simulink model "robot_2015"  (R2015b)
(part 17 of 148)

  Cylindrical9/LConn1 -- hex_bolt_gradeb_iso_243_RIGID/RConn1
  Cylindrical9/RConn1 -- hex_nut_style_1_gradeab_iso_156_RIGID/LConn2
  Cylindrical10/LConn1 -- hex_bolt_gradeb_iso_247_RIGID/RConn1
  Cylindrical10/RConn1 -- hex_nut_style_1_gradeab_iso_158_RIGID/LConn2
  Cylindrical11/LConn1 -- hex_bolt_gradeb_iso_209_RIGID/RConn1
  Planar3/LConn1 -- hip_joint_casin_2_RIGID/RConn5
  Cylindrical11/RConn1 -- hex_nut_style_1_gradeab_iso_161_RIGID/LConn2
  Cylindrical12/LConn1 -- hex_bolt_gradeb_iso_211_RIGID/RConn1
  Cylindrical12/RConn1 -- hex_nut_style_1_gradeab_iso_162_RIGID/LConn1
  Cylindrical13/LConn1 -- hex_bolt_gradeb_iso_208_RIGID/RConn1
  Cylindrical13/RConn1 -- hex_nut_style_1_gradeab_iso_163_RIGID/LConn2
  Cylindrical14/LConn1 -- hex_bolt_gradeb_iso_249_RIGID/RConn1
  Cylindrical14/RConn1 -- hex_nut_style_1_gradeab_iso_164_RIGID/LConn2
  Cylindrical15/LConn1 -- hex_bolt_gradeb_iso_254_RIGID/RConn1
  Cylindrical15/RConn1 -- hex_nut_style_1_gradeab_iso_165_RIGID/LConn2
  Cylindrical16/LConn1 -- hex_bolt_gradeb_iso_253_RIGID/RConn1
  Planar3/RConn1 -- hex_nut_style_1_gradeab_iso_258_RIGID/LConn2
  Cylindrical16/RConn1 -- hex_nut_style_1_gradeab_iso_166_RIGID/LConn1
  Cylindrical17/LConn1 -- hex_bolt_gradeb_iso_210_RIGID/RConn1
  Cylindrical17/RConn1 -- hex_nut_style_1_gradeab_iso_167_RIGID/LConn2
  Cylindrical18/LConn1 -- hex_bolt_gradeb_iso_252_RIGID/RConn1
  Cylindrical18/RConn1 -- hex_nut_style_1_gradeab_iso_168_RIGID/LConn1
  Cylindrical19/LConn1 -- hex_bolt_gradeb_iso_251_RIGID/RConn1
  Cylindrical19/RConn1 -- hex_nut_style_1_gradeab_iso_169_RIGID/LConn2
  Cylindrical20/LConn1 -- hex_bolt_gradeb_iso_250_RIGID/RConn1
  Cylindrical20/RConn1 -- hex_nut_style_1_gradeab_iso_170_RIGID/LConn2
  Cylindrical21/LConn1 -- hex_bolt_gradeb_iso_206_RIGID/RConn1
  Planar4/LConn1 -- hip_joint_casin_2_RIGID/RConn3
  Cylindrical21/RConn1 -- hex_nut_style_1_gradeab_iso_171_RIGID/LConn1
  Cylindrical22/LConn1 -- hex_bolt_gradeb_iso_207_RIGID/RConn1
  Cylindrical22/RConn1 -- hex_nut_style_1_gradeab_iso_172_RIGID/LConn1
  Cylindrical23/LConn1 -- hex_bolt_gradeb_iso_220_RIGID/RConn1
  Cylindrical23/RConn1 -- hex_nut_style_1_gradeab_iso_185_RIGID/LConn1
  Cylindrical24/LConn1 -- hex_bolt_gradeb_iso_221_RIGID/RConn1
  Cylindrical24/RConn1 -- hex_nut_style_1_gradeab_iso_186_RIGID/LConn2
  Cylindrical25/LConn1 -- hex_bolt_gradeb_iso_222_RIGID/RConn1
  Cylindrical25/RConn1 -- hex_nut_style_1_gradeab_iso_187_RIGID/LConn2
  Cylindrical26/LConn1 -- hex_bolt_gradeb_iso_223_RIGID/RConn1
  Planar4/RConn1 -- hex_nut_style_1_gradeab_iso_259_RIGID/LConn2
  Cylindrical26/RConn1 -- hex_nut_style_1_gradeab_iso_188_RIGID/LConn2
  Cylindrical27/LConn1 -- hex_bolt_gradeb_iso_218_RIGID/RConn1
  Cylindrical27/RConn1 -- hex_nut_style_1_gradeab_iso_189_RIGID/LConn1
  Cylindrical28/LConn1 -- hex_bolt_gradeb_iso_219_RIGID/RConn1
  Cylindrical28/RConn1 -- hex_nut_style_1_gradeab_iso_190_RIGID/LConn1
  Cylindrical29/LConn1 -- hex_bolt_gradeb_iso_257_RIGID/RConn1
  Cylindrical29/RConn1 -- hex_nut_style_1_gradeab_iso_191_RIGID/LConn2
  Cylindrical30/LConn1 -- hex_bolt_gradeb_iso_258_RIGID/RConn1
  Cylindrical30/RConn1 -- hex_nut_style_1_gradeab_iso_192_RIGID/LConn2
  Cylindrical31/LConn1 -- hex_bolt_gradeb_iso_259_RIGID/RConn1
  Revolute1/RConn1 -- hex_nut_style_1_gradeab_iso_249_RIGID/LConn1
  Planar5/LConn1 -- hip_joint_casin_2_RIGID/RConn6
  Cylindrical31/RConn1 -- hex_nut_style_1_gradeab_iso_193_RIGID/LConn2
  Cylindrical32/LConn1 -- hex_bolt_gradeb_iso_260_RIGID/RConn1
  Cylindrical32/RConn1 -- hex_nut_style_1_gradeab_iso_194_RIGID/LConn2
  Cylindrical33/LConn1 -- hex_bolt_gradeb_iso_255_RIGID/RConn1
  Cylindrical33/RConn1 -- hex_nut_style_1_gradeab_iso_195_RIGID/LConn1
  Cylindrical34/LConn1 -- hex_bolt_gradeb_iso_256_RIGID/RConn1
  Cylindrical34/RConn1 -- hex_nut_style_1_gradeab_iso_196_RIGID/LConn1
  Cylindrical35/LConn1 -- hex_bolt_gradeb_iso_235_RIGID/RConn1
  Cylindrical35/RConn1 -- hex_nut_style_1_gradeab_iso_197_RIGID/LConn1
  Cylindrical36/LConn1 -- hex_bolt_gradeb_iso_230_RIGID/RConn1
  Planar5/RConn1 -- hex_nut_style_1_gradeab_iso_260_RIGID/LConn1
  Cylindrical36/RConn1 -- hex_nut_style_1_gradeab_iso_199_RIGID/LConn2
  Cylindrical37/LConn1 -- hex_bolt_gradeb_iso_234_RIGID/RConn1
  Cylindrical37/RConn1 -- hex_nut_style_1_gradeab_iso_201_RIGID/LConn1
  Cylindrical38/LConn1 -- hex_bolt_gradeb_iso_233_RIGID/RConn1
  Cylindrical38/RConn1 -- hex_nut_style_1_gradeab_iso_204_RIGID/LConn2
  Cylindrical39/LConn1 -- hex_bolt_gradeb_iso_232_RIGID/RConn1
  Cylindrical39/RConn1 -- hex_nut_style_1_gradeab_iso_205_RIGID/LConn1
  Cylindrical40/LConn1 -- hex_bolt_gradeb_iso_231_RIGID/RConn1
  Cylindrical40/RConn1 -- hex_nut_style_1_gradeab_iso_206_RIGID/LConn1
  Cylindrical41/LConn1 -- hex_bolt_gradeb_iso_268_RIGID/RConn1
  Revolute14/LConn1 -- hip_joint_casin_2_RIGID/RConn2
  Cylindrical41/RConn1 -- hex_nut_style_1_gradeab_iso_215_RIGID/LConn2
  Cylindrical42/LConn1 -- hex_bolt_gradeb_iso_267_RIGID/RConn1
  Cylindrical42/RConn1 -- hex_nut_style_1_gradeab_iso_216_RIGID/LConn1
  Cylindrical43/LConn1 -- hex_bolt_gradeb_iso_271_RIGID/RConn1
  Cylindrical43/RConn1 -- hex_nut_style_1_gradeab_iso_217_RIGID/LConn2
  Cylindrical44/LConn1 -- hex_bolt_gradeb_iso_272_RIGID/RConn1
  Cylindrical44/RConn1 -- hex_nut_style_1_gradeab_iso_218_RIGID/LConn1
  Cylindrical45/LConn1 -- hex_bolt_gradeb_iso_270_RIGID/RConn1
  Cylindrical45/RConn1 -- hex_nut_style_1_gradeab_iso_219_RIGID/LConn1
  Cylindrical46/LConn1 -- hex_bolt_gradeb_iso_269_RIGID/RConn1
  Revolute14/RConn1 -- hex_bolt_gradeb_iso_206_RIGID/LConn1
  Cylindrical46/RConn1 -- hex_nut_style_1_gradeab_iso_220_RIGID/LConn2
  Cylindrical47/LConn1 -- hex_bolt_gradeb_iso_160_RIGID/RConn1
  Cylindrical47/RConn1 -- hex_nut_style_1_gradeab_iso_222_RIGID/LConn1
  Cylindrical48/LConn1 -- hex_bolt_gradeb_iso_161_RIGID/RConn1
  Cylindrical48/RConn1 -- hex_nut_style_1_gradeab_iso_223_RIGID/LConn1
  Cylindrical49/LConn1 -- hex_bolt_gradeb_iso_162_RIGID/RConn1
  Cylindrical49/RConn1 -- hex_nut_style_1_gradeab_iso_224_RIGID/LConn1
  Cylindrical50/LConn1 -- hex_bolt_gradeb_iso_157_RIGID/RConn1
  Cylindrical50/RConn1 -- hex_nut_style_1_gradeab_iso_225_RIGID/LConn1
  Cylindrical51/LConn1 -- hex_bolt_gradeb_iso_158_RIGID/RConn1
  Revolute15/LConn1 -- hip_joint_casin_2_RIGID/RConn1
  Cylindrical51/RConn1 -- hex_nut_style_1_gradeab_iso_226_RIGID/LConn1
  Cylindrical52/LConn1 -- hex_bolt_gradeb_iso_159_RIGID/RConn1
  Cylindrical52/RConn1 -- hex_nut_style_1_gradeab_iso_227_RIGID/LConn1
  Cylindrical53/LConn1 -- hex_bolt_gradeb_iso_171_RIGID/RConn1
  Cylindrical53/RConn1 -- hex_nut_style_1_gradeab_iso_240_RIGID/LConn2
  Cylindrical54/LConn1 -- hex_bolt_gradeb_iso_170_RIGID/RConn1
  Cylindrical54/RConn1 -- hex_nut_style_1_gradeab_iso_241_RIGID/LConn2
  Cylindrical55/LConn1 -- hex_bolt_gradeb_iso_174_RIGID/RConn1
  Cylindrical55/RConn1 -- hex_nut_style_1_gradeab_iso_242_RIGID/LConn1
  Cylindrical56/LConn1 -- hex_bolt_gradeb_iso_173_RIGID/RConn1
  Revolute15/RConn1 -- hex_bolt_gradeb_iso_207_RIGID/LConn1
  Cylindrical56/RConn1 -- hex_nut_style_1_gradeab_iso_243_RIGID/LConn2
  Cylindrical57/LConn1 -- hex_bolt_gradeb_iso_172_RIGID/RConn1
  Cylindrical57/RConn1 -- hex_nut_style_1_gradeab_iso_244_RIGID/LConn1
  Cylindrical58/LConn1 -- hex_bolt_gradeb_iso_169_RIGID/RConn1
  Cylindrical58/RConn1 -- hex_nut_style_1_gradeab_iso_248_RIGID/LConn2
  Cylindrical59/LConn1 -- hex_bolt_gradeb_iso_147_RIGID/RConn1
  Cylindrical59/RConn1 -- hex_nut_style_1_gradeab_iso_255_RIGID/LConn1
  Cylindrical60/LConn1 -- hex_bolt_gradeb_iso_148_RIGID/RConn1
  Cylindrical60/RConn1 -- hex_nut_style_1_gradeab_iso_256_RIGID/LConn2
  Cylindrical61/LConn1 -- hex_bolt_gradeb_iso_146_RIGID/RConn1
  Revolute16/LConn1 -- hip_joint_casin_2_RIGID/RConn12
  Cylindrical61/RConn1 -- hex_nut_style_1_gradeab_iso_257_RIGID/LConn2
  Cylindrical62/LConn1 -- hex_bolt_gradeb_iso_150_RIGID/RConn1
  Cylindrical62/RConn1 -- hex_nut_style_1_gradeab_iso_258_RIGID/LConn1
  Cylindrical63/LConn1 -- hex_bolt_gradeb_iso_149_RIGID/RConn1
  Cylindrical63/RConn1 -- hex_nut_style_1_gradeab_iso_259_RIGID/LConn1
  Cylindrical64/LConn1 -- hex_bolt_gradeb_iso_145_RIGID/RConn1
  Cylindrical64/RConn1 -- hex_nut_style_1_gradeab_iso_260_RIGID/LConn2
  Cylindrical65/LConn1 -- hex_bolt_gradeb_iso_181_RIGID/RConn1
  Cylindrical65/RConn1 -- hex_nut_style_1_gradeab_iso_267_RIGID/LConn2
  Cylindrical66/LConn1 -- hex_bolt_gradeb_iso_184_RIGID/RConn1
  Revolute16/RConn1 -- hex_bolt_gradeb_iso_208_RIGID/LConn1
  Cylindrical66/RConn1 -- hex_nut_style_1_gradeab_iso_268_RIGID/LConn1
  Cylindrical67/LConn1 -- hex_bolt_gradeb_iso_185_RIGID/RConn1
  Cylindrical67/RConn1 -- hex_nut_style_1_gradeab_iso_269_RIGID/LConn1
  Cylindrical68/LConn1 -- hex_bolt_gradeb_iso_186_RIGID/RConn1
  Cylindrical68/RConn1 -- hex_nut_style_1_gradeab_iso_270_RIGID/LConn1
  Cylindrical69/LConn1 -- hex_bolt_gradeb_iso_182_RIGID/RConn1
  Cylindrical69/RConn1 -- hex_nut_style_1_gradeab_iso_271_RIGID/LConn1
  Cylindrical70/LConn1 -- hex_bolt_gradeb_iso_183_RIGID/RConn1
  Cylindrical70/RConn1 -- hex_nut_style_1_gradeab_iso_272_RIGID/LConn1
  Cylindrical71/LConn1 -- hex_bolt_gradeb_iso_195_RIGID/RConn1
  Revolute17/LConn1 -- hip_joint_casin_2_RIGID/RConn11
  Cylindrical71/RConn1 -- hex_nut_style_1_gradeab_iso_279_RIGID/LConn1
  Cylindrical72/LConn1 -- hex_bolt_gradeb_iso_194_RIGID/RConn1
  Cylindrical72/RConn1 -- hex_nut_style_1_gradeab_iso_280_RIGID/LConn2
  Cylindrical73/LConn1 -- hex_bolt_gradeb_iso_193_RIGID/RConn1
  Cylindrical73/RConn1 -- hex_nut_style_1_gradeab_iso_281_RIGID/LConn2
  Cylindrical74/LConn1 -- hex_bolt_gradeb_iso_198_RIGID/RConn1
  Cylindrical74/RConn1 -- hex_nut_style_1_gradeab_iso_282_RIGID/LConn1
  Cylindrical75/LConn1 -- hex_bolt_gradeb_iso_197_RIGID/RConn1
  Cylindrical75/RConn1 -- hex_nut_style_1_gradeab_iso_283_RIGID/LConn1
  Cylindrical76/LConn1 -- hex_bolt_gradeb_iso_196_RIGID/RConn1
  Revolute17/RConn1 -- hex_bolt_gradeb_iso_209_RIGID/LConn1
  Cylindrical76/RConn1 -- hex_nut_style_1_gradeab_iso_284_RIGID/LConn1
  Rectangular1/LConn1 -- SEA_system_1_RIGID/RConn1
  Rectangular1/RConn1 -- lower_leg_main_1_RIGID/LConn2
  Revolute111/LConn1 -- lower_leg_main_1_RIGID/RConn12
  Revolute111/RConn1 -- hex_bolt_gradeb_iso_193_RIGID/LConn1
  Revolute112/LConn1 -- lower_leg_main_1_RIGID/RConn10
  Revolute112/RConn1 -- hex_bolt_gradeb_iso_194_RIGID/LConn1
  Revolute113/LConn1 -- lower_leg_main_1_RIGID/RConn7
  Revolute113/RConn1 -- hex_bolt_gradeb_iso_195_RIGID/LConn1
  Revolute114/LConn1 -- lower_leg_main_1_RIGID/RConn6
  Revolute2/LConn1 -- hip_joint_casin_1_RIGID/RConn7
  Revolute18/LConn1 -- hip_joint_casin_2_RIGID/RConn10
  Revolute114/RConn1 -- hex_bolt_gradeb_iso_196_RIGID/LConn1
  Revolute115/LConn1 -- lower_leg_main_1_RIGID/RConn5
  Revolute115/RConn1 -- hex_bolt_gradeb_iso_197_RIGID/LConn1
  Revolute116/LConn1 -- lower_leg_main_1_RIGID/RConn4
  Revolute116/RConn1 -- hex_bolt_gradeb_iso_198_RIGID/LConn1
  Revolute117/LConn1 -- lower_leg_main_1_RIGID/RConn3
  Revolute117/RConn1 -- hex_bolt_gradeb_iso_199_RIGID/LConn1
  Revolute118/LConn1 -- lower_leg_main_1_RIGID/RConn2
  Revolute118/RConn1 -- hex_bolt_gradeb_iso_200_RIGID/LConn1
  Revolute119/LConn1 -- lower_leg_main_1_RIGID/RConn1
  Revolute18/RConn1 -- hex_bolt_gradeb_iso_210_RIGID/LConn1
  Revolute119/RConn1 -- hex_bolt_gradeb_iso_201_RIGID/LConn1
  Revolute120/LConn1 -- lower_leg_main_1_RIGID/RConn11
  Revolute120/RConn1 -- hex_bolt_gradeb_iso_202_RIGID/LConn1
  Revolute121/LConn1 -- lower_leg_main_1_RIGID/RConn9
  Revolute121/RConn1 -- hex_bolt_gradeb_iso_203_RIGID/LConn1
  Revolute122/LConn1 -- lower_leg_main_1_RIGID/RConn8
  Revolute122/RConn1 -- hex_bolt_gradeb_iso_204_RIGID/LConn1
  Cylindrical77/LConn1 -- motor_axle_1_RIGID/RConn2
  Cylindrical77/RConn1 -- upper_leg_casin_2_RIGID/LConn2
  Revolute123/LConn1 -- motor_body_1_RIGID/RConn1
  Revolute19/LConn1 -- hip_joint_casin_2_RIGID/RConn8
  Revolute123/RConn1 -- upper_leg_casin_2_RIGID/LConn3
  Revolute124/LConn1 -- upper_leg_casin_2_RIGID/RConn7
  Revolute124/RConn1 -- hex_bolt_gradeb_iso_243_RIGID/LConn1
  Revolute125/LConn1 -- upper_leg_casin_2_RIGID/RConn6
  Revolute125/RConn1 -- hex_bolt_gradeb_iso_244_RIGID/LConn1
  Revolute126/LConn1 -- upper_leg_casin_2_RIGID/RConn5
  Revolute126/RConn1 -- hex_bolt_gradeb_iso_245_RIGID/LConn1
  Revolute127/LConn1 -- upper_leg_casin_2_RIGID/RConn4
  Revolute127/RConn1 -- hex_bolt_gradeb_iso_246_RIGID/LConn1
  Revolute128/LConn1 -- upper_leg_casin_2_RIGID/RConn3
  Revolute19/RConn1 -- hex_bolt_gradeb_iso_211_RIGID/LConn1
  Revolute128/RConn1 -- hex_bolt_gradeb_iso_247_RIGID/LConn1
  Revolute129/LConn1 -- upper_leg_casin_2_RIGID/RConn2
  Revolute129/RConn1 -- hex_bolt_gradeb_iso_248_RIGID/LConn1
  Prismatic4/LConn1 -- upper_leg_casin_2_RIGID/RConn1
  Prismatic4/RConn1 -- upper_leg_cap_7_RIGID/LConn2
  motor_body_2_RIGID/LConn1 -- upper_leg_casin_3_RIGID/LConn4
  Planar44/LConn1 -- upper_leg_casin_3_RIGID/RConn8
  Planar44/RConn1 -- hex_nut_style_1_gradeab_iso_222_RIGID/LConn2
  Planar45/LConn1 -- upper_leg_casin_3_RIGID/RConn7
  Planar45/RConn1 -- hex_nut_style_1_gradeab_iso_223_RIGID/LConn2
  Lower_joint_cap_1_RIGID/RConn6 -- Revolute20/LConn1
  Planar46/LConn1 -- upper_leg_casin_3_RIGID/RConn6
  Planar46/RConn1 -- hex_nut_style_1_gradeab_iso_224_RIGID/LConn2
  Planar47/LConn1 -- upper_leg_casin_3_RIGID/RConn5
  Planar47/RConn1 -- hex_nut_style_1_gradeab_iso_225_RIGID/LConn2
  Planar48/LConn1 -- upper_leg_casin_3_RIGID/RConn4
  Planar48/RConn1 -- hex_nut_style_1_gradeab_iso_226_RIGID/LConn2
  Planar49/LConn1 -- upper_leg_casin_3_RIGID/RConn3
  Planar49/RConn1 -- hex_nut_style_1_gradeab_iso_227_RIGID/LConn2
  Revolute130/LConn1 -- upper_leg_casin_3_RIGID/RConn2
  Revolute130/RConn1 -- hex_bolt_gradeb_iso_261_RIGID/LConn1
  Revolute20/RConn1 -- hex_nut_style_1_gradeab_iso_145_RIGID/LConn1
  Revolute131/LConn1 -- upper_leg_casin_3_RIGID/RConn1
  Revolute131/RConn1 -- hex_bolt_gradeb_iso_262_RIGID/LConn1
  Revolute132/LConn1 -- upper_leg_casin_3_RIGID/RConn12
  Revolute132/RConn1 -- hex_bolt_gradeb_iso_263_RIGID/LConn1
  Revolute133/LConn1 -- upper_leg_casin_3_RIGID/RConn11
  Revolute133/RConn1 -- hex_bolt_gradeb_iso_264_RIGID/LConn1
  Revolute134/LConn1 -- upper_leg_casin_3_RIGID/RConn10
  Revolute134/RConn1 -- hex_bolt_gradeb_iso_265_RIGID/LConn1
  Revolute135/LConn1 -- upper_leg_casin_3_RIGID/RConn9
  Revolute135/RConn1 -- hex_bolt_gradeb_iso_266_RIGID/LConn1
  Lower_joint_cap_1_RIGID/RConn5 -- Revolute21/LConn1
  Prismatic5/LConn1 -- upper_leg_cap_3_RIGID/RConn1
  Prismatic5/RConn1 -- upper_leg_casin_3_RIGID/LConn2
  Revolute136/LConn1 -- upper_leg_casin_4_RIGID/RConn11
  Revolute136/RConn1 -- hex_nut_style_1_gradeab_iso_228_RIGID/LConn1
  Revolute137/LConn1 -- upper_leg_casin_4_RIGID/RConn8
  Revolute137/RConn1 -- hex_nut_style_1_gradeab_iso_230_RIGID/LConn1
  Revolute138/LConn1 -- upper_leg_casin_4_RIGID/RConn7
  Revolute138/RConn1 -- hex_nut_style_1_gradeab_iso_231_RIGID/LConn1
  Revolute139/LConn1 -- upper_leg_casin_4_RIGID/RConn6
  Revolute139/RConn1 -- hex_nut_style_1_gradeab_iso_232_RIGID/LConn1
  Revolute21/RConn1 -- hex_nut_style_1_gradeab_iso_146_RIGID/LConn1
  Revolute140/LConn1 -- upper_leg_casin_4_RIGID/RConn5
  Revolute140/RConn1 -- hex_nut_style_1_gradeab_iso_233_RIGID/LConn1
  Revolute141/LConn1 -- upper_leg_casin_4_RIGID/RConn4
  Revolute141/RConn1 -- hex_bolt_gradeb_iso_255_RIGID/LConn1
  Revolute142/LConn1 -- upper_leg_casin_4_RIGID/RConn1
  Revolute142/RConn1 -- hex_bolt_gradeb_iso_256_RIGID/LConn1
  Revolute143/LConn1 -- upper_leg_casin_4_RIGID/RConn3
  Revolute143/RConn1 -- hex_bolt_gradeb_iso_257_RIGID/LConn1
  Revolute144/LConn1 -- upper_leg_casin_4_RIGID/RConn2
  Revolute144/RConn1 -- hex_bolt_gradeb_iso_258_RIGID/LConn1
  Lower_joint_cap_1_RIGID/RConn4 -- Revolute22/LConn1
  Revolute145/LConn1 -- upper_leg_casin_4_RIGID/RConn10
  Revolute145/RConn1 -- hex_bolt_gradeb_iso_259_RIGID/LConn1
  Revolute146/LConn1 -- upper_leg_casin_4_RIGID/RConn9
  Revolute146/RConn1 -- hex_bolt_gradeb_iso_260_RIGID/LConn1
  Prismatic6/LConn1 -- upper_leg_cap_4_RIGID/RConn1
  Prismatic6/RConn1 -- upper_leg_casin_4_RIGID/LConn2
  Cylindrical78/LConn1 -- motor_axle_3_RIGID/RConn2
  Cylindrical78/RConn1 -- upper_leg_casin_5_RIGID/LConn3
  Revolute147/LConn1 -- motor_body_3_RIGID/RConn1
  Revolute147/RConn1 -- upper_leg_casin_5_RIGID/LConn4
  Revolute22/RConn1 -- hex_nut_style_1_gradeab_iso_147_RIGID/LConn1
  upper_leg_casin_5_RIGID/LConn1 -- upperleg_1_RIGID/LConn5
  Planar50/LConn1 -- upper_leg_casin_5_RIGID/RConn5
  Planar50/RConn1 -- hex_nut_style_1_gradeab_iso_267_RIGID/LConn1
  Planar51/LConn1 -- upper_leg_casin_5_RIGID/RConn4
  Planar51/RConn1 -- hex_nut_style_1_gradeab_iso_268_RIGID/LConn2
  Planar52/LConn1 -- upper_leg_casin_5_RIGID/RConn3
  Planar52/RConn1 -- hex_nut_style_1_gradeab_iso_269_RIGID/LConn2
  Planar53/LConn1 -- upper_leg_casin_5_RIGID/RConn2
  Planar53/RConn1 -- hex_nut_style_1_gradeab_iso_270_RIGID/LConn2
  Planar54/LConn1 -- upper_leg_casin_5_RIGID/RConn1
  Revolute2/RConn1 -- hex_nut_style_1_gradeab_iso_250_RIGID/LConn1
  Lower_joint_cap_1_RIGID/RConn3 -- Revolute23/LConn1
  Planar54/RConn1 -- hex_nut_style_1_gradeab_iso_271_RIGID/LConn2
  Planar55/LConn1 -- upper_leg_casin_5_RIGID/RConn8
  Planar55/RConn1 -- hex_nut_style_1_gradeab_iso_272_RIGID/LConn2
  Revolute148/LConn1 -- upper_leg_casin_5_RIGID/RConn12
  Revolute148/RConn1 -- hex_bolt_gradeb_iso_273_RIGID/LConn1
  Revolute149/LConn1 -- upper_leg_casin_5_RIGID/RConn11
  Revolute149/RConn1 -- hex_bolt_gradeb_iso_274_RIGID/LConn1
  Revolute150/LConn1 -- upper_leg_casin_5_RIGID/RConn10
  Revolute150/RConn1 -- hex_bolt_gradeb_iso_275_RIGID/LConn1
  Revolute151/LConn1 -- upper_leg_casin_5_RIGID/RConn9
  Revolute23/RConn1 -- hex_nut_style_1_gradeab_iso_150_RIGID/LConn1
  Revolute151/RConn1 -- hex_bolt_gradeb_iso_276_RIGID/LConn1
  Revolute152/LConn1 -- upper_leg_casin_5_RIGID/RConn7
  Revolute152/RConn1 -- hex_bolt_gradeb_iso_277_RIGID/LConn1
  Revolute153/LConn1 -- upper_leg_casin_5_RIGID/RConn6
  Revolute153/RConn1 -- hex_bolt_gradeb_iso_278_RIGID/LConn1
  upper_leg_casin_6_RIGID/LConn1 -- upperleg_1_RIGID/LConn4
  Revolute154/LConn1 -- upper_leg_casin_6_RIGID/RConn10
  Revolute154/RConn1 -- hex_nut_style_1_gradeab_iso_261_RIGID/LConn1
  Revolute155/LConn1 -- upper_leg_casin_6_RIGID/RConn9
  Revolute155/RConn1 -- hex_nut_style_1_gradeab_iso_262_RIGID/LConn1
  Lower_joint_cap_1_RIGID/RConn2 -- Revolute24/LConn1
  Revolute156/LConn1 -- upper_leg_casin_6_RIGID/RConn7
  Revolute156/RConn1 -- hex_nut_style_1_gradeab_iso_263_RIGID/LConn1
  Revolute157/LConn1 -- upper_leg_casin_6_RIGID/RConn6
  Revolute157/RConn1 -- hex_nut_style_1_gradeab_iso_264_RIGID/LConn1
  Revolute158/LConn1 -- upper_leg_casin_6_RIGID/RConn5
  Revolute158/RConn1 -- hex_nut_style_1_gradeab_iso_265_RIGID/LConn1
  Revolute159/LConn1 -- upper_leg_casin_6_RIGID/RConn4
  Revolute159/RConn1 -- hex_nut_style_1_gradeab_iso_266_RIGID/LConn1
  Revolute160/LConn1 -- upper_leg_casin_6_RIGID/RConn1
  Revolute160/RConn1 -- hex_bolt_gradeb_iso_267_RIGID/LConn1
  Revolute24/RConn1 -- hex_nut_style_1_gradeab_iso_159_RIGID/LConn1
  Revolute161/LConn1 -- upper_leg_casin_6_RIGID/RConn13
  Revolute161/RConn1 -- hex_bolt_gradeb_iso_268_RIGID/LConn1
  Revolute162/LConn1 -- upper_leg_casin_6_RIGID/RConn12
  Revolute162/RConn1 -- hex_bolt_gradeb_iso_269_RIGID/LConn1
  Revolute163/LConn1 -- upper_leg_casin_6_RIGID/RConn2
  Revolute163/RConn1 -- hex_bolt_gradeb_iso_270_RIGID/LConn1
  Revolute164/LConn1 -- upper_leg_casin_6_RIGID/RConn11
  Revolute164/RConn1 -- hex_bolt_gradeb_iso_271_RIGID/LConn1
  Revolute165/LConn1 -- upper_leg_casin_6_RIGID/RConn3
  Revolute165/RConn1 -- hex_bolt_gradeb_iso_272_RIGID/LConn1
  Lower_joint_cap_1_RIGID/RConn1 -- Revolute25/LConn1
  Revolute166/LConn1 -- upper_leg_casin_7_RIGID/RConn6
  Revolute166/RConn1 -- hex_bolt_gradeb_iso_249_RIGID/LConn1
  Revolute167/LConn1 -- upper_leg_casin_7_RIGID/RConn5
  Revolute167/RConn1 -- hex_bolt_gradeb_iso_250_RIGID/LConn1
  Revolute168/LConn1 -- upper_leg_casin_7_RIGID/RConn4
  Revolute168/RConn1 -- hex_bolt_gradeb_iso_251_RIGID/LConn1
  Revolute169/LConn1 -- upper_leg_casin_7_RIGID/RConn3
  Revolute169/RConn1 -- hex_bolt_gradeb_iso_252_RIGID/LConn1
  Revolute170/LConn1 -- upper_leg_casin_7_RIGID/RConn1
  Revolute170/RConn1 -- hex_bolt_gradeb_iso_253_RIGID/LConn1
  Revolute25/RConn1 -- hex_nut_style_1_gradeab_iso_160_RIGID/LConn1
  Revolute171/LConn1 -- upper_leg_casin_7_RIGID/RConn2
  Revolute171/RConn1 -- hex_bolt_gradeb_iso_254_RIGID/LConn1
  Prismatic7/LConn1 -- upper_leg_cap_1_RIGID/RConn2
  Prismatic7/RConn1 -- upper_leg_casin_7_RIGID/LConn2
  Prismatic8/LConn1 -- motor_axle_1_RIGID/RConn1
  Prismatic8/RConn1 -- SEA_system_hip_1_RIGID/LConn2
  Rectangular2/LConn1 -- hip_1_RIGID/RConn25
  Rectangular2/RConn1 -- SEA_system_hip_1_RIGID/LConn1
  Lower_joint_casin_1_RIGID/RConn12 -- Prismatic9/LConn1
  Prismatic9/RConn1 -- beam_filler_1_RIGID/LConn1
  Ball_bearing_filler_2_RIGID/LConn1 -- Lower_joint_cap_1_RIGID/LConn1
  beam_filler_1_RIGID/LConn2 -- upperleg_1_RIGID/LConn3
  Lower_joint_casin_2_RIGID/LConn2 -- beam_filler_2_RIGID/LConn1
  beam_filler_2_RIGID/LConn2 -- upperleg_1_RIGID/LConn1
  Lower_joint_casin_5_RIGID/LConn3 -- beam_filler_3_RIGID/LConn1
  beam_filler_3_RIGID/LConn2 -- lower_leg_main_1_RIGID/LConn1
  Revolute172/LConn1 -- beam_filler_4_RIGID/RConn2
  Lower_joint_casin_3_RIGID/LConn2 -- Revolute172/RConn1
  Prismatic10/LConn1 -- beam_filler_4_RIGID/RConn1
  Prismatic10/RConn1 -- lower_leg_main_1_RIGID/LConn3
  Planar56/LConn1 -- upper_leg_cap_1_RIGID/RConn1
  Lower_joint_cap_2_RIGID/RConn6 -- Planar6/LConn1
  Planar56/RConn1 -- bearing_1_RIGID/LConn1
  Ball_bearing_filler_small_1_RIGID/LConn2 -- upper_leg_cap_1_RIGID/LConn1
  Planar57/LConn1 -- upper_leg_cap_2_RIGID/RConn6
  Planar57/RConn1 -- hex_nut_style_1_gradeab_iso_164_RIGID/LConn1
  Planar58/LConn1 -- upper_leg_cap_2_RIGID/RConn5
  Planar58/RConn1 -- hex_nut_style_1_gradeab_iso_165_RIGID/LConn1
  Planar59/LConn1 -- upper_leg_cap_2_RIGID/RConn2
  Planar59/RConn1 -- hex_nut_style_1_gradeab_iso_166_RIGID/LConn2
  Planar60/LConn1 -- upper_leg_cap_2_RIGID/RConn1
  Planar60/RConn1 -- hex_nut_style_1_gradeab_iso_168_RIGID/LConn2
  Planar6/RConn1 -- hex_nut_style_1_gradeab_iso_161_RIGID/LConn1
  Planar61/LConn1 -- upper_leg_cap_2_RIGID/RConn4
  Planar61/RConn1 -- hex_nut_style_1_gradeab_iso_169_RIGID/LConn1
  Planar62/LConn1 -- upper_leg_cap_2_RIGID/RConn3
  Planar62/RConn1 -- hex_nut_style_1_gradeab_iso_170_RIGID/LConn1
  Ball_bearing_filler_small_1_RIGID/LConn1 -- upper_leg_cap_2_RIGID/LConn1
  Revolute173/LConn1 -- bearing_3_RIGID/RConn1
  Revolute173/RConn1 -- upper_leg_cap_3_RIGID/LConn2
  Ball_bearing_filler_small_4_RIGID/LConn2 -- upper_leg_cap_3_RIGID/LConn1
  Revolute174/LConn1 -- upper_leg_cap_4_RIGID/RConn2
  Revolute174/RConn1 -- bearing_4_RIGID/LConn1
  Lower_joint_cap_2_RIGID/RConn3 -- Planar7/LConn1
  Ball_bearing_filler_small_3_RIGID/LConn2 -- upper_leg_cap_4_RIGID/LConn1
  Revolute175/LConn1 -- upper_leg_cap_5_RIGID/RConn6
  Revolute175/RConn1 -- hex_nut_style_1_gradeab_iso_198_RIGID/LConn1
  Revolute176/LConn1 -- upper_leg_cap_5_RIGID/RConn5
  Revolute176/RConn1 -- hex_nut_style_1_gradeab_iso_200_RIGID/LConn1
  Revolute177/LConn1 -- upper_leg_cap_5_RIGID/RConn4
  Revolute177/RConn1 -- hex_nut_style_1_gradeab_iso_202_RIGID/LConn1
  Revolute178/LConn1 -- upper_leg_cap_5_RIGID/RConn3
  Revolute178/RConn1 -- hex_nut_style_1_gradeab_iso_203_RIGID/LConn1
  Revolute179/LConn1 -- upper_leg_cap_5_RIGID/RConn2
  Revolute3/LConn1 -- hip_joint_casin_1_RIGID/RConn6
  Planar7/RConn1 -- hex_nut_style_1_gradeab_iso_162_RIGID/LConn2
  Revolute179/RConn1 -- hex_nut_style_1_gradeab_iso_207_RIGID/LConn1
  Revolute180/LConn1 -- upper_leg_cap_5_RIGID/RConn1
  Revolute180/RConn1 -- hex_nut_style_1_gradeab_iso_208_RIGID/LConn1
  Ball_bearing_filler_small_6_RIGID/LConn1 -- upper_leg_cap_5_RIGID/LConn1
  Planar63/LConn1 -- upper_leg_cap_6_RIGID/RConn6
  Planar63/RConn1 -- hex_nut_style_1_gradeab_iso_215_RIGID/LConn1
  Planar64/LConn1 -- upper_leg_cap_6_RIGID/RConn3
  Planar64/RConn1 -- hex_nut_style_1_gradeab_iso_216_RIGID/LConn2
  Planar65/LConn1 -- upper_leg_cap_6_RIGID/RConn5
  Planar65/RConn1 -- hex_nut_style_1_gradeab_iso_217_RIGID/LConn1
  Lower_joint_cap_2_RIGID/RConn5 -- Planar8/LConn1
  Planar66/LConn1 -- upper_leg_cap_6_RIGID/RConn2
  Planar66/RConn1 -- hex_nut_style_1_gradeab_iso_218_RIGID/LConn2
  Planar67/LConn1 -- upper_leg_cap_6_RIGID/RConn1
  Planar67/RConn1 -- hex_nut_style_1_gradeab_iso_219_RIGID/LConn2
  Planar68/LConn1 -- upper_leg_cap_6_RIGID/RConn4
  Planar68/RConn1 -- hex_nut_style_1_gradeab_iso_220_RIGID/LConn1
  Ball_bearing_filler_small_5_RIGID/LConn2 -- upper_leg_cap_6_RIGID/LConn1
  Planar69/LConn1 -- bearing_2_RIGID/RConn2
  Planar69/RConn1 -- upper_leg_cap_7_RIGID/LConn1
  Ball_bearing_filler_small_2_RIGID/LConn1 -- upper_leg_cap_7_RIGID/LConn3
  Planar8/RConn1 -- hex_nut_style_1_gradeab_iso_163_RIGID/LConn1
  Planar70/LConn1 -- upper_leg_cap_8_RIGID/RConn6
  Planar70/RConn1 -- hex_nut_style_1_gradeab_iso_151_RIGID/LConn1
  Planar71/LConn1 -- upper_leg_cap_8_RIGID/RConn5
  Planar71/RConn1 -- hex_nut_style_1_gradeab_iso_152_RIGID/LConn1
  Planar72/LConn1 -- upper_leg_cap_8_RIGID/RConn4
  Planar72/RConn1 -- hex_nut_style_1_gradeab_iso_153_RIGID/LConn1
  Planar73/LConn1 -- upper_leg_cap_8_RIGID/RConn2
  Planar73/RConn1 -- hex_nut_style_1_gradeab_iso_154_RIGID/LConn2
  Planar74/LConn1 -- upper_leg_cap_8_RIGID/RConn3
  Planar74/RConn1 -- hex_nut_style_1_gradeab_iso_156_RIGID/LConn1
  Lower_joint_cap_2_RIGID/RConn4 -- Planar9/LConn1
  Planar75/LConn1 -- upper_leg_cap_8_RIGID/RConn1
  Planar75/RConn1 -- hex_nut_style_1_gradeab_iso_158_RIGID/LConn1
  Ball_bearing_filler_small_2_RIGID/LConn3 -- upper_leg_cap_8_RIGID/LConn1
  Planar76/LConn1 -- upper_leg_cap_9_RIGID/RConn6
  Planar76/RConn1 -- hex_nut_style_1_gradeab_iso_191_RIGID/LConn1
  Planar77/LConn1 -- upper_leg_cap_9_RIGID/RConn4
  Planar77/RConn1 -- hex_nut_style_1_gradeab_iso_192_RIGID/LConn1
  Planar78/LConn1 -- upper_leg_cap_9_RIGID/RConn5
  Planar78/RConn1 -- hex_nut_style_1_gradeab_iso_193_RIGID/LConn1
  Planar79/LConn1 -- upper_leg_cap_9_RIGID/RConn3
  Planar9/RConn1 -- hex_nut_style_1_gradeab_iso_167_RIGID/LConn1
  Planar79/RConn1 -- hex_nut_style_1_gradeab_iso_194_RIGID/LConn1
  Planar80/LConn1 -- upper_leg_cap_9_RIGID/RConn2
  Planar80/RConn1 -- hex_nut_style_1_gradeab_iso_195_RIGID/LConn2
  Planar81/LConn1 -- upper_leg_cap_9_RIGID/RConn1
  Planar81/RConn1 -- hex_nut_style_1_gradeab_iso_196_RIGID/LConn2
  Ball_bearing_filler_small_3_RIGID/LConn1 -- upper_leg_cap_9_RIGID/LConn1
  Revolute181/LConn1 -- hip_joint_casin_2_RIGID/RConn4
  Ball_bearing_filler_1_RIGID/LConn2 -- Revolute181/RConn1
  Cylindrical79/LConn1 -- bearing_1_RIGID/RConn2
  Ball_bearing_filler_1_RIGID/LConn1 -- Cylindrical79/RConn1
  Lower_joint_cap_2_RIGID/RConn2 -- Planar10/LConn1
  Revolute182/LConn1 -- hip_joint_casin_1_RIGID/RConn9
  Ball_bearing_filler_2_RIGID/LConn2 -- Revolute182/RConn1
  Cylindrical80/LConn1 -- bearing_2_RIGID/RConn1
  Ball_bearing_filler_2_RIGID/LConn3 -- Cylindrical80/RConn1
  Ball_bearing_filler_3_RIGID/LConn2 -- Lower_joint_casin_2_RIGID/LConn1
  Ball_bearing_filler_4_RIGID/LConn2 -- Lower_joint_casin_1_RIGID/LConn1
  Ball_bearing_filler_5_RIGID/LConn1 -- Lower_joint_casin_3_RIGID/LConn1
  Ball_bearing_filler_6_RIGID/RConn1 -- Revolute183/LConn1
  Lower_joint_casin_5_RIGID/LConn1 -- Revolute183/RConn1
  Cylindrical81/LConn1 -- bearing_6_RIGID/RConn1
  Planar10/RConn1 -- hex_nut_style_1_gradeab_iso_171_RIGID/LConn2
  Ball_bearing_filler_6_RIGID/LConn1 -- Cylindrical81/RConn1
  beam_filler_hip_1_RIGID/LConn1 -- hip_1_RIGID/LConn4
  beam_filler_hip_2_RIGID/LConn2 -- hip_1_RIGID/LConn1
  Revolute184/LConn1 -- hip_1_RIGID/RConn6
  Revolute184/RConn1 -- hex_bolt_gradeb_iso_145_RIGID/LConn1
  Revolute185/LConn1 -- hip_1_RIGID/RConn5
  Revolute185/RConn1 -- hex_bolt_gradeb_iso_146_RIGID/LConn1
  Revolute186/LConn1 -- hip_1_RIGID/RConn7
  Revolute186/RConn1 -- hex_bolt_gradeb_iso_147_RIGID/LConn1
  Revolute187/LConn1 -- hip_1_RIGID/RConn4
  Lower_joint_cap_2_RIGID/RConn1 -- Planar11/LConn1
  Revolute187/RConn1 -- hex_bolt_gradeb_iso_148_RIGID/LConn1
  Revolute188/LConn1 -- hip_1_RIGID/RConn2
  Revolute188/RConn1 -- hex_bolt_gradeb_iso_149_RIGID/LConn1
  Revolute189/LConn1 -- hip_1_RIGID/RConn3
  Revolute189/RConn1 -- hex_bolt_gradeb_iso_150_RIGID/LConn1
  Revolute190/LConn1 -- hip_1_RIGID/RConn1
  Revolute190/RConn1 -- hex_bolt_gradeb_iso_151_RIGID/LConn1
  Revolute191/LConn1 -- hip_1_RIGID/RConn24
  Revolute191/RConn1 -- hex_bolt_gradeb_iso_152_RIGID/LConn1
  Revolute192/LConn1 -- hip_1_RIGID/RConn23
  Planar11/RConn1 -- hex_nut_style_1_gradeab_iso_172_RIGID/LConn2
  Revolute192/RConn1 -- hex_bolt_gradeb_iso_153_RIGID/LConn1
  Revolute193/LConn1 -- hip_1_RIGID/RConn22
  Revolute193/RConn1 -- hex_bolt_gradeb_iso_154_RIGID/LConn1
  Revolute194/LConn1 -- hip_1_RIGID/RConn21
  Revolute194/RConn1 -- hex_bolt_gradeb_iso_155_RIGID/LConn1
  Revolute195/LConn1 -- hip_1_RIGID/RConn20
  Revolute195/RConn1 -- hex_bolt_gradeb_iso_156_RIGID/LConn1
  Revolute196/LConn1 -- hip_1_RIGID/RConn19
  Revolute196/RConn1 -- hex_bolt_gradeb_iso_157_RIGID/LConn1
  Revolute197/LConn1 -- hip_1_RIGID/RConn18
  Ball_bearing_filler_1_RIGID/LConn3 -- Lower_joint_cap_2_RIGID/LConn1
  Revolute197/RConn1 -- hex_bolt_gradeb_iso_158_RIGID/LConn1
  Revolute198/LConn1 -- hip_1_RIGID/RConn16
  Revolute198/RConn1 -- hex_bolt_gradeb_iso_159_RIGID/LConn1
  Revolute199/LConn1 -- hip_1_RIGID/RConn17
  Revolute199/RConn1 -- hex_bolt_gradeb_iso_160_RIGID/LConn1
  Revolute200/LConn1 -- hip_1_RIGID/RConn15
  Revolute200/RConn1 -- hex_bolt_gradeb_iso_161_RIGID/LConn1
  Revolute201/LConn1 -- hip_1_RIGID/RConn14
  Revolute201/RConn1 -- hex_bolt_gradeb_iso_162_RIGID/LConn1
  Revolute202/LConn1 -- hip_1_RIGID/RConn13
  Revolute3/RConn1 -- hex_nut_style_1_gradeab_iso_251_RIGID/LConn1
  Lower_joint_cap_3_RIGID/RConn6 -- Revolute26/LConn1
  Revolute202/RConn1 -- hex_bolt_gradeb_iso_163_RIGID/LConn1
  Revolute203/LConn1 -- hip_1_RIGID/RConn12
  Revolute203/RConn1 -- hex_bolt_gradeb_iso_164_RIGID/LConn1
  Revolute204/LConn1 -- hip_1_RIGID/RConn11
  Revolute204/RConn1 -- hex_bolt_gradeb_iso_165_RIGID/LConn1
  Revolute205/LConn1 -- hip_1_RIGID/RConn10
  Revolute205/RConn1 -- hex_bolt_gradeb_iso_166_RIGID/LConn1
  Revolute206/LConn1 -- hip_1_RIGID/RConn9
  Revolute206/RConn1 -- hex_bolt_gradeb_iso_167_RIGID/LConn1
  Revolute207/LConn1 -- hip_1_RIGID/RConn8
  Revolute26/RConn1 -- hex_nut_style_1_gradeab_iso_173_RIGID/LConn1
  Revolute207/RConn1 -- hex_bolt_gradeb_iso_168_RIGID/LConn1
  hip_1_RIGID/LConn3 -- upper_leg_casin_3_RIGID/LConn1
  hip_1_RIGID/LConn2 -- upper_leg_casin_4_RIGID/LConn1
  upper_leg_casin_2_RIGID/LConn4 -- F/RConn1
  upper_leg_casin_7_RIGID/LConn1 -- F1/RConn1
  Lower_joint_cap_3_RIGID/RConn5 -- Revolute27/LConn1
  Revolute27/RConn1 -- hex_nut_style_1_gradeab_iso_174_RIGID/LConn1
  Lower_joint_cap_3_RIGID/RConn4 -- Revolute28/LConn1
  Revolute28/RConn1 -- hex_nut_style_1_gradeab_iso_177_RIGID/LConn1
  Lower_joint_cap_3_RIGID/RConn3 -- Revolute29/LConn1
  Revolute29/RConn1 -- hex_nut_style_1_gradeab_iso_180_RIGID/LConn1
  Lower_joint_cap_3_RIGID/RConn2 -- Revolute30/LConn1
  Revolute30/RConn1 -- hex_nut_style_1_gradeab_iso_181_RIGID/LConn1
  Revolute4/LConn1 -- hip_joint_casin_1_RIGID/RConn5
  Lower_joint_cap_3_RIGID/RConn1 -- Revolute31/LConn1
  Revolute31/RConn1 -- hex_nut_style_1_gradeab_iso_184_RIGID/LConn1
  Ball_bearing_filler_4_RIGID/LConn1 -- Lower_joint_cap_3_RIGID/LConn1
  Lower_joint_cap_4_RIGID/RConn4 -- Planar12/LConn1
  Planar12/RConn1 -- hex_nut_style_1_gradeab_iso_185_RIGID/LConn2
  Lower_joint_cap_4_RIGID/RConn6 -- Planar13/LConn1
  Planar13/RConn1 -- hex_nut_style_1_gradeab_iso_186_RIGID/LConn1
  Lower_joint_cap_4_RIGID/RConn5 -- Planar14/LConn1
  Planar14/RConn1 -- hex_nut_style_1_gradeab_iso_187_RIGID/LConn1
  Lower_joint_cap_4_RIGID/RConn3 -- Planar15/LConn1
  "rightLegController "/RConn1 -- Revolute44/LConn2
  "rightLegController "/RConn2 -- Revolute45/LConn2
  "rightLegController "/RConn3 -- Revolute46/LConn2
  "rightLegController "/LConn1 -- Revolute44/RConn2
  "rightLegController "/LConn6 -- Revolute46/RConn3
  "rightLegController "/LConn5 -- Revolute46/RConn2
  "rightLegController "/LConn4 -- Revolute45/RConn3
  "rightLegController "/LConn3 -- Revolute45/RConn2
  "rightLegController "/LConn2 -- Revolute44/RConn3
